simulink model "CLIK_con_trasposta"  (R2022b)
settings: Solver=VariableStepAuto  StartTime=0.0  StopTime=40  RelTol=1e-3
values from neighbouring files (symbols this model uses):
  k_trasposta = 500    [CLIK_script.m]
  T = T_A * T_B    [DH_dinamica.m]    (also in traiettoria_script.m = 0.001)
  theta1_0 = pi/2 - angolo    [CLIK_script.m]
  theta2_0 = 2*angolo    [CLIK_script.m]
undefined symbols (not defined in the file or in its folder): DiscIntNeverNeededParam
libraries: simulink x1
settings Model: Creator=Michele  LastModifiedBy=Michele
settings DataIOCC: ReturnWorkspaceOutputs=off

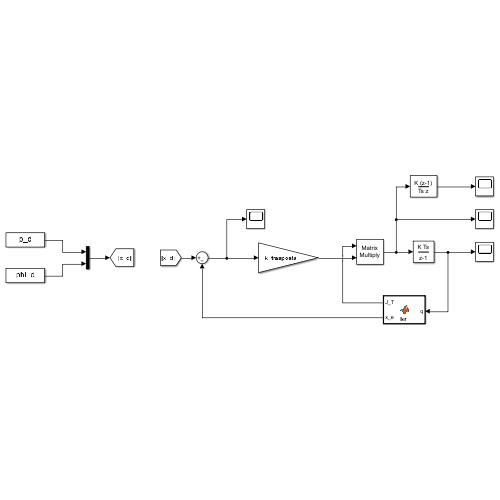
[thumbnail: Simulink's stored preview of the top-level diagram]
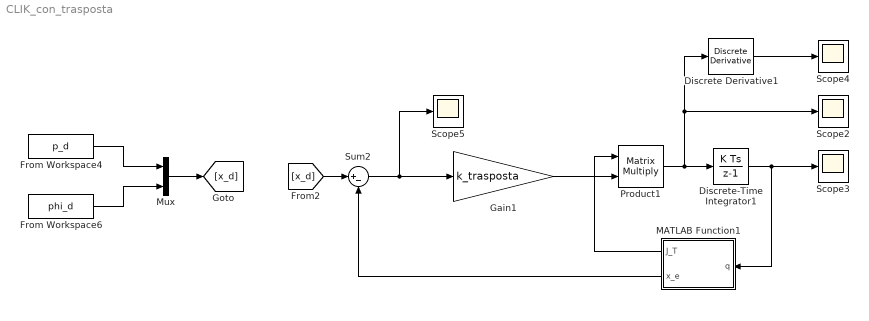
== system CLIK_con_trasposta ==
  Discrete Derivative1 : simulink/Discrete/Discrete Derivative  gainval=1.0  ICPrevScaledInput=[0 0 0 0]'  OutMin=[]  OutMax=[]  OutDataType=fixdt(1, 16)  OutScaling=2^-10  DoSatur=off
  Discrete-Time Integrator1 : DiscreteIntegrator  InitialCondition=[theta1_0 theta2_0 -0.25 0]'  SampleTime=-1  ICPrevOutput=DiscIntNeverNeededParam  ICPrevScaledInput=DiscIntNeverNeededParam
  From Workspace4 : FromWorkspace  VariableName=p_d  SampleTime=T
  From Workspace6 : FromWorkspace  VariableName=phi_d  SampleTime=T
  Gain1 : Gain  Gain=k_trasposta
  MATLAB Function1 : MATLAB Function  TreatAsAtomicUnit=on
  Mux : Mux  Inputs=2
  Product1 : Product  Multiplication=Matrix(*)
  Scope{2..5} (4 alike) : Scope
  Sum2 : Sum  Inputs=|+-
  wires:
  Product1/1 -> Discrete-Time Integrator1/1, Discrete Derivative1/1, Scope2/1
  Discrete-Time Integrator1/1 -> MATLAB Function1/1(q), Scope3/1
  Gain1/1 -> Product1/2
  MATLAB Function1/2(x_e) -> Sum2/2
  MATLAB Function1/1(J_T) -> Product1/1
  Discrete Derivative1/1 -> Scope4/1
  [x_d] -> Sum2/1
  Sum2/1 -> Scope5/1, Gain1/1
  Mux/1 -> [x_d]
  From Workspace4/1 -> Mux/1
  From Workspace6/1 -> Mux/2

== matlab function CLIK_con_trasposta/MATLAB Function1 ==
  data: J_T output; q input; x_e output
function [J_T,x_e] = kin(q)

    q1 = q(1); q2 = q(2); q3 = q(3); q4 = q(4);

    J = [- sin(q1)/2 - (cos(q1)*sin(q2))/2 - (cos(q2)*sin(q1))/2, - (cos(q1)*sin(q2))/2 - (cos(q2)*sin(q1))/2, 0, 0;
           cos(q1)/2 + (cos(q1)*cos(q2))/2 - (sin(q1)*sin(q2))/2,   (cos(q1)*cos(q2))/2 - (sin(q1)*sin(q2))/2, 0, 0;
                                                               0,                                           0, 1, 0;
                                                               0,                                           0, 0, 1];

    x_e = [cos(q1)/2 + (cos(q1)*cos(q2))/2 - (sin(q1)*sin(q2))/2;
           sin(q1)/2 + (cos(q1)*sin(q2))/2 + (cos(q2)*sin(q1))/2;
                                                   q3;
                                                   q4];

    J_T = transpose(J);
end
